simulink model "platoon1"  (R2023a)
settings: Solver=ode2  StartTime=0.0  StopTime=20  FixedStep=1/600  RelTol=1e-3  EnableMultiTasking=on
undefined symbols (not defined in the file or in its folder): HIL, qc_get_step_size
libraries: simulink x29, quarc_library x29, slpidlib x27, cstblocks x23, eeStairGenerator x1
(part 3 of 4)

== system platoon1/Controller8 ==
  PosPred : Inport
  PosEgo : Inport  Port=2
  d_ref : Inport  Port=3
  PosLead : Inport  Port=4
  i : Inport  Port=5
  Add : Sum  Inputs=+-
  Add1 : Sum  Inputs=-+
  Add2 : Sum
  Add3 : Sum  Inputs=+-
  Add4 : Sum  Inputs=-+
  Integrator : Integrator
  PID Controller : slpidlib/PID Controller  Controller=PID  Form=Parallel  TimeDomain=Continuous-time  UseExternalTs=off  SampleTime=-1  IntegratorMethod=Forward Euler  FilterMethod=Forward Euler  ControllerParametersSource=internal  P=0.33095280227445  I=0.0676054764431606  UseKiTs=off  D=0.347839718693587  N=40.6182647095365  UseFilter=on  TunerSelectOption=Transfer Function Based (PID Tuner App)  InitialConditionSource=internal  InitialConditionForIntegrator=0  InitialConditionForFilter=0  DifferentiatorICPrevScaledInput=0  ExternalReset=none  TrackingMode=off  Kt=1  LimitOutput=off  SatLimitsSource=internal  UpperSaturationLimit=inf  LowerSaturationLimit=-inf  LinearizeAsGain=on  AntiWindupMode=none  Kb=1  LimitIntegrator=off  UpperIntegratorSaturationLimit=inf  LowerIntegratorSaturationLimit=-inf  POutMin=[]  POutMax=[]  IOutMin=[]  IOutMax=[]  DOutMin=[]  DOutMax=[]  NOutMin=[]  NOutMax=[]  SumOutMin=[]  SumOutMax=[]  SaturationOutMin=[]  SaturationOutMax=[]  PParamMin=[]  PParamMax=[]  IParamMin=[]  IParamMax=[]  DParamMin=[]  DParamMax=[]  NParamMin=[]  NParamMax=[]  KbParamMin=[]  KbParamMax=[]  KtParamMin=[]  KtParamMax=[]  KbOutMin=[]  KbOutMax=[]  KtOutMin=[]  KtOutMax=[]  IntegratorOutMin=[]  IntegratorOutMax=[]  FilterOutMin=[]  FilterOutMax=[]  SumI1OutMin=[]  SumI1OutMax=[]  SumI2OutMin=[]  SumI2OutMax=[]  SumI3OutMin=[]  SumI3OutMax=[]  SumI4OutMin=[]  SumI4OutMax=[]  SumDOutMin=[]  SumDOutMax=[]  DifferentiatorOutMin=[]  DifferentiatorOutMax=[]  FilterDiffOutCoefMin=[]  FilterDiffOutCoefMax=[]  ReciprocalOutMin=[]  ReciprocalOutMax=[]  SumDenOutMin=[]  SumDenOutMax=[]  SumNumOutMin=[]  SumNumOutMax=[]  DivideOutMin=[]  DivideOutMax=[]  UdiffTsProdOutMin=[]  UdiffTsProdOutMax=[]  NTsProdOutMin=[]  NTsProdOutMax=[]  UintegralTsProdOutMin=[]  UintegralTsProdOutMax=[]  UngainTsProdOutMin=[]  UngainTsProdOutMax=[]  ClampingZeroOutDataTypeStr=Inherit: Inherit via back propagation  ClampingZeroOutMin=[]  ClampingZeroOutMax=[]  FilterDenConstantOutDataTypeStr=Inherit: Inherit via back propagation  FilterDenConstantOutMin=[]  FilterDenConstantOutMax=[]  PCopyOutDataTypeStr=Inherit: Inherit via back propagation  PCopyOutMin=[]  PCopyOutMax=[]  NCopyOutDataTypeStr=Inherit: Inherit via back propagation  NCopyOutMin=[]  NCopyOutMax=[]  IntegratorContinuousStateAttributes=''  IntegratorStateMustResolveToSignalObject=off  IntegratorRTWStateStorageClass=Auto  FilterContinuousStateAttributes=''  FilterStateMustResolveToSignalObject=off  FilterRTWStateStorageClass=Auto  ParallelPVariant=InternalParameters  IdealPVariant=Disabled  IVariant=InternalParameters  DVariant=InternalParameters  IntegratorVariant=Continuous  SatVariant=Disabled  AWVariant=Passthrough  PCopyVariant=Disabled  TRVariant=Disabled  FdbkBlocksVariant=Forward  IdealPFdbkVariant=Disabled  SatFdbkVariant=Disabled  DerivativeFilterVariant=ContFilter  NVariant=InternalParameters  NCopyVariant=Disabled  FilterICVariant=InternalICsFilter  IntegratorICVariant=InternalICs  ExternalResetVariant=Disabled  TRSumVariant=Passthrough  SumFdbkVariant=Disabled  SumVariant=Sum_PID  TsampFilterVariant=InternalTs  TsampNgainVariant=Passthrough  TsampIntegralVariant=Disabled_SignalSpec  ExternalSaturationOutDataTypeStr=Inherit: Same as second input
  PID Controller1 : slpidlib/PID Controller  Controller=PID  Form=Parallel  TimeDomain=Continuous-time  UseExternalTs=off  SampleTime=-1  IntegratorMethod=Forward Euler  FilterMethod=Forward Euler  ControllerParametersSource=internal  P=0.0689075408458366  I=0.00109879069900871  UseKiTs=off  D=0.960150912828831  N=312.36902011058  UseFilter=on  TunerSelectOption=Transfer Function Based (PID Tuner App)  InitialConditionSource=internal  InitialConditionForIntegrator=0  InitialConditionForFilter=0  DifferentiatorICPrevScaledInput=0  ExternalReset=none  TrackingMode=off  Kt=1  LimitOutput=off  SatLimitsSource=internal  UpperSaturationLimit=inf  LowerSaturationLimit=-inf  LinearizeAsGain=on  AntiWindupMode=none  Kb=1  LimitIntegrator=off  UpperIntegratorSaturationLimit=inf  LowerIntegratorSaturationLimit=-inf  POutMin=[]  POutMax=[]  IOutMin=[]  IOutMax=[]  DOutMin=[]  DOutMax=[]  NOutMin=[]  NOutMax=[]  SumOutMin=[]  SumOutMax=[]  SaturationOutMin=[]  SaturationOutMax=[]  PParamMin=[]  PParamMax=[]  IParamMin=[]  IParamMax=[]  DParamMin=[]  DParamMax=[]  NParamMin=[]  NParamMax=[]  KbParamMin=[]  KbParamMax=[]  KtParamMin=[]  KtParamMax=[]  KbOutMin=[]  KbOutMax=[]  KtOutMin=[]  KtOutMax=[]  IntegratorOutMin=[]  IntegratorOutMax=[]  FilterOutMin=[]  FilterOutMax=[]  SumI1OutMin=[]  SumI1OutMax=[]  SumI2OutMin=[]  SumI2OutMax=[]  SumI3OutMin=[]  SumI3OutMax=[]  SumI4OutMin=[]  SumI4OutMax=[]  SumDOutMin=[]  SumDOutMax=[]  DifferentiatorOutMin=[]  DifferentiatorOutMax=[]  FilterDiffOutCoefMin=[]  FilterDiffOutCoefMax=[]  ReciprocalOutMin=[]  ReciprocalOutMax=[]  SumDenOutMin=[]  SumDenOutMax=[]  SumNumOutMin=[]  SumNumOutMax=[]  DivideOutMin=[]  DivideOutMax=[]  UdiffTsProdOutMin=[]  UdiffTsProdOutMax=[]  NTsProdOutMin=[]  NTsProdOutMax=[]  UintegralTsProdOutMin=[]  UintegralTsProdOutMax=[]  UngainTsProdOutMin=[]  UngainTsProdOutMax=[]  ClampingZeroOutDataTypeStr=Inherit: Inherit via back propagation  ClampingZeroOutMin=[]  ClampingZeroOutMax=[]  FilterDenConstantOutDataTypeStr=Inherit: Inherit via back propagation  FilterDenConstantOutMin=[]  FilterDenConstantOutMax=[]  PCopyOutDataTypeStr=Inherit: Inherit via back propagation  PCopyOutMin=[]  PCopyOutMax=[]  NCopyOutDataTypeStr=Inherit: Inherit via back propagation  NCopyOutMin=[]  NCopyOutMax=[]  IntegratorContinuousStateAttributes=''  IntegratorStateMustResolveToSignalObject=off  IntegratorRTWStateStorageClass=Auto  FilterContinuousStateAttributes=''  FilterStateMustResolveToSignalObject=off  FilterRTWStateStorageClass=Auto  ParallelPVariant=InternalParameters  IdealPVariant=Disabled  IVariant=InternalParameters  DVariant=InternalParameters  IntegratorVariant=Continuous  SatVariant=Disabled  AWVariant=Passthrough  PCopyVariant=Disabled  TRVariant=Disabled  FdbkBlocksVariant=Forward  IdealPFdbkVariant=Disabled  SatFdbkVariant=Disabled  DerivativeFilterVariant=ContFilter  NVariant=InternalParameters  NCopyVariant=Disabled  FilterICVariant=InternalICsFilter  IntegratorICVariant=InternalICs  ExternalResetVariant=Disabled  TRSumVariant=Passthrough  SumFdbkVariant=Disabled  SumVariant=Sum_PID  TsampFilterVariant=InternalTs  TsampNgainVariant=Passthrough  TsampIntegralVariant=Disabled_SignalSpec  ExternalSaturationOutDataTypeStr=Inherit: Same as second input
  Product : Product
  Speed : Outport
  wires:
  PosPred/1 -> Add/1
  PosEgo/1 -> Add/2, Add3/2
  Add/1 -> Add1/2  "d_act"
  d_ref/1 -> Product/2, Add1/1
  Add1/1 -> PID Controller/1  "d_error_pred"
  Add2/1 -> Integrator/1
  PID Controller/1 -> Add2/2
  PosLead/1 -> Add3/1
  Add3/1 -> Add4/2  "d_act"
  Product/1 -> Add4/1
  i/1 -> Product/1
  Add4/1 -> PID Controller1/1  "d_error_lead"
  PID Controller1/1 -> Add2/1
  Integrator/1 -> Speed/1

== system platoon1/Controller9 ==
  PosPred : Inport
  PosEgo : Inport  Port=2
  d_ref : Inport  Port=3
  PosLead : Inport  Port=4
  i : Inport  Port=5
  Add : Sum  Inputs=+-
  Add1 : Sum  Inputs=-+
  Add2 : Sum
  Add3 : Sum  Inputs=+-
  Add4 : Sum  Inputs=-+
  Integrator : Integrator
  PID Controller : slpidlib/PID Controller  Controller=PID  Form=Parallel  TimeDomain=Continuous-time  UseExternalTs=off  SampleTime=-1  IntegratorMethod=Forward Euler  FilterMethod=Forward Euler  ControllerParametersSource=internal  P=0.33095280227445  I=0.0676054764431606  UseKiTs=off  D=0.347839718693587  N=40.6182647095365  UseFilter=on  TunerSelectOption=Transfer Function Based (PID Tuner App)  InitialConditionSource=internal  InitialConditionForIntegrator=0  InitialConditionForFilter=0  DifferentiatorICPrevScaledInput=0  ExternalReset=none  TrackingMode=off  Kt=1  LimitOutput=off  SatLimitsSource=internal  UpperSaturationLimit=inf  LowerSaturationLimit=-inf  LinearizeAsGain=on  AntiWindupMode=none  Kb=1  LimitIntegrator=off  UpperIntegratorSaturationLimit=inf  LowerIntegratorSaturationLimit=-inf  POutMin=[]  POutMax=[]  IOutMin=[]  IOutMax=[]  DOutMin=[]  DOutMax=[]  NOutMin=[]  NOutMax=[]  SumOutMin=[]  SumOutMax=[]  SaturationOutMin=[]  SaturationOutMax=[]  PParamMin=[]  PParamMax=[]  IParamMin=[]  IParamMax=[]  DParamMin=[]  DParamMax=[]  NParamMin=[]  NParamMax=[]  KbParamMin=[]  KbParamMax=[]  KtParamMin=[]  KtParamMax=[]  KbOutMin=[]  KbOutMax=[]  KtOutMin=[]  KtOutMax=[]  IntegratorOutMin=[]  IntegratorOutMax=[]  FilterOutMin=[]  FilterOutMax=[]  SumI1OutMin=[]  SumI1OutMax=[]  SumI2OutMin=[]  SumI2OutMax=[]  SumI3OutMin=[]  SumI3OutMax=[]  SumI4OutMin=[]  SumI4OutMax=[]  SumDOutMin=[]  SumDOutMax=[]  DifferentiatorOutMin=[]  DifferentiatorOutMax=[]  FilterDiffOutCoefMin=[]  FilterDiffOutCoefMax=[]  ReciprocalOutMin=[]  ReciprocalOutMax=[]  SumDenOutMin=[]  SumDenOutMax=[]  SumNumOutMin=[]  SumNumOutMax=[]  DivideOutMin=[]  DivideOutMax=[]  UdiffTsProdOutMin=[]  UdiffTsProdOutMax=[]  NTsProdOutMin=[]  NTsProdOutMax=[]  UintegralTsProdOutMin=[]  UintegralTsProdOutMax=[]  UngainTsProdOutMin=[]  UngainTsProdOutMax=[]  ClampingZeroOutDataTypeStr=Inherit: Inherit via back propagation  ClampingZeroOutMin=[]  ClampingZeroOutMax=[]  FilterDenConstantOutDataTypeStr=Inherit: Inherit via back propagation  FilterDenConstantOutMin=[]  FilterDenConstantOutMax=[]  PCopyOutDataTypeStr=Inherit: Inherit via back propagation  PCopyOutMin=[]  PCopyOutMax=[]  NCopyOutDataTypeStr=Inherit: Inherit via back propagation  NCopyOutMin=[]  NCopyOutMax=[]  IntegratorContinuousStateAttributes=''  IntegratorStateMustResolveToSignalObject=off  IntegratorRTWStateStorageClass=Auto  FilterContinuousStateAttributes=''  FilterStateMustResolveToSignalObject=off  FilterRTWStateStorageClass=Auto  ParallelPVariant=InternalParameters  IdealPVariant=Disabled  IVariant=InternalParameters  DVariant=InternalParameters  IntegratorVariant=Continuous  SatVariant=Disabled  AWVariant=Passthrough  PCopyVariant=Disabled  TRVariant=Disabled  FdbkBlocksVariant=Forward  IdealPFdbkVariant=Disabled  SatFdbkVariant=Disabled  DerivativeFilterVariant=ContFilter  NVariant=InternalParameters  NCopyVariant=Disabled  FilterICVariant=InternalICsFilter  IntegratorICVariant=InternalICs  ExternalResetVariant=Disabled  TRSumVariant=Passthrough  SumFdbkVariant=Disabled  SumVariant=Sum_PID  TsampFilterVariant=InternalTs  TsampNgainVariant=Passthrough  TsampIntegralVariant=Disabled_SignalSpec  ExternalSaturationOutDataTypeStr=Inherit: Same as second input
  PID Controller1 : slpidlib/PID Controller  Controller=PID  Form=Parallel  TimeDomain=Continuous-time  UseExternalTs=off  SampleTime=-1  IntegratorMethod=Forward Euler  FilterMethod=Forward Euler  ControllerParametersSource=internal  P=0.0689075408458366  I=0.00109879069900871  UseKiTs=off  D=0.960150912828831  N=312.36902011058  UseFilter=on  TunerSelectOption=Transfer Function Based (PID Tuner App)  InitialConditionSource=internal  InitialConditionForIntegrator=0  InitialConditionForFilter=0  DifferentiatorICPrevScaledInput=0  ExternalReset=none  TrackingMode=off  Kt=1  LimitOutput=off  SatLimitsSource=internal  UpperSaturationLimit=inf  LowerSaturationLimit=-inf  LinearizeAsGain=on  AntiWindupMode=none  Kb=1  LimitIntegrator=off  UpperIntegratorSaturationLimit=inf  LowerIntegratorSaturationLimit=-inf  POutMin=[]  POutMax=[]  IOutMin=[]  IOutMax=[]  DOutMin=[]  DOutMax=[]  NOutMin=[]  NOutMax=[]  SumOutMin=[]  SumOutMax=[]  SaturationOutMin=[]  SaturationOutMax=[]  PParamMin=[]  PParamMax=[]  IParamMin=[]  IParamMax=[]  DParamMin=[]  DParamMax=[]  NParamMin=[]  NParamMax=[]  KbParamMin=[]  KbParamMax=[]  KtParamMin=[]  KtParamMax=[]  KbOutMin=[]  KbOutMax=[]  KtOutMin=[]  KtOutMax=[]  IntegratorOutMin=[]  IntegratorOutMax=[]  FilterOutMin=[]  FilterOutMax=[]  SumI1OutMin=[]  SumI1OutMax=[]  SumI2OutMin=[]  SumI2OutMax=[]  SumI3OutMin=[]  SumI3OutMax=[]  SumI4OutMin=[]  SumI4OutMax=[]  SumDOutMin=[]  SumDOutMax=[]  DifferentiatorOutMin=[]  DifferentiatorOutMax=[]  FilterDiffOutCoefMin=[]  FilterDiffOutCoefMax=[]  ReciprocalOutMin=[]  ReciprocalOutMax=[]  SumDenOutMin=[]  SumDenOutMax=[]  SumNumOutMin=[]  SumNumOutMax=[]  DivideOutMin=[]  DivideOutMax=[]  UdiffTsProdOutMin=[]  UdiffTsProdOutMax=[]  NTsProdOutMin=[]  NTsProdOutMax=[]  UintegralTsProdOutMin=[]  UintegralTsProdOutMax=[]  UngainTsProdOutMin=[]  UngainTsProdOutMax=[]  ClampingZeroOutDataTypeStr=Inherit: Inherit via back propagation  ClampingZeroOutMin=[]  ClampingZeroOutMax=[]  FilterDenConstantOutDataTypeStr=Inherit: Inherit via back propagation  FilterDenConstantOutMin=[]  FilterDenConstantOutMax=[]  PCopyOutDataTypeStr=Inherit: Inherit via back propagation  PCopyOutMin=[]  PCopyOutMax=[]  NCopyOutDataTypeStr=Inherit: Inherit via back propagation  NCopyOutMin=[]  NCopyOutMax=[]  IntegratorContinuousStateAttributes=''  IntegratorStateMustResolveToSignalObject=off  IntegratorRTWStateStorageClass=Auto  FilterContinuousStateAttributes=''  FilterStateMustResolveToSignalObject=off  FilterRTWStateStorageClass=Auto  ParallelPVariant=InternalParameters  IdealPVariant=Disabled  IVariant=InternalParameters  DVariant=InternalParameters  IntegratorVariant=Continuous  SatVariant=Disabled  AWVariant=Passthrough  PCopyVariant=Disabled  TRVariant=Disabled  FdbkBlocksVariant=Forward  IdealPFdbkVariant=Disabled  SatFdbkVariant=Disabled  DerivativeFilterVariant=ContFilter  NVariant=InternalParameters  NCopyVariant=Disabled  FilterICVariant=InternalICsFilter  IntegratorICVariant=InternalICs  ExternalResetVariant=Disabled  TRSumVariant=Passthrough  SumFdbkVariant=Disabled  SumVariant=Sum_PID  TsampFilterVariant=InternalTs  TsampNgainVariant=Passthrough  TsampIntegralVariant=Disabled_SignalSpec  ExternalSaturationOutDataTypeStr=Inherit: Same as second input
  Product : Product
  Speed : Outport
  wires:
  PosPred/1 -> Add/1
  PosEgo/1 -> Add/2, Add3/2
  Add/1 -> Add1/2  "d_act"
  d_ref/1 -> Product/2, Add1/1
  Add1/1 -> PID Controller/1  "d_error_pred"
  Add2/1 -> Integrator/1
  PID Controller/1 -> Add2/2
  PosLead/1 -> Add3/1
  Add3/1 -> Add4/2  "d_act"
  Product/1 -> Add4/1
  i/1 -> Product/1
  Add4/1 -> PID Controller1/1  "d_error_lead"
  PID Controller1/1 -> Add2/1
  Integrator/1 -> Speed/1

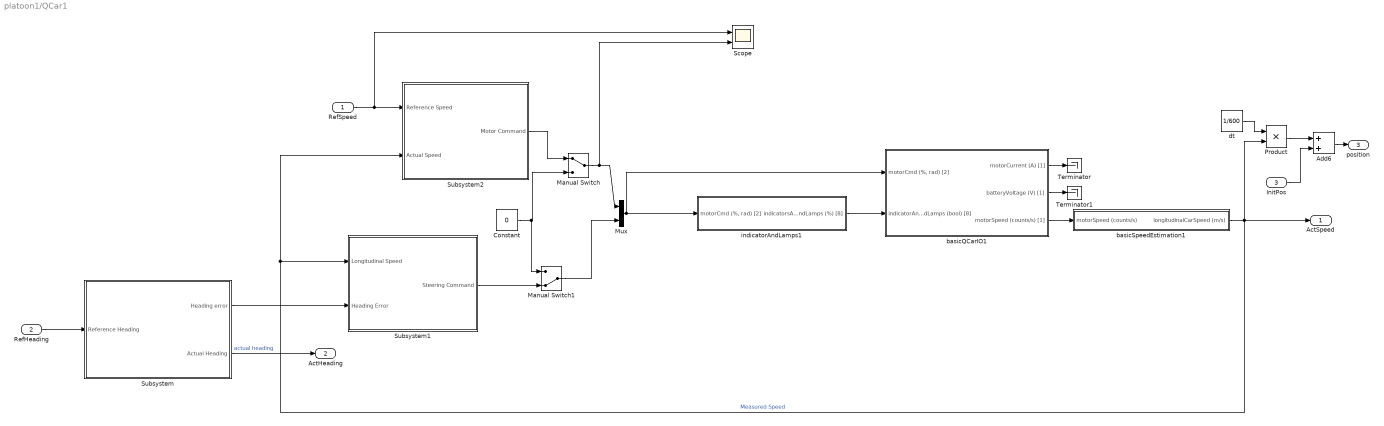
== system platoon1/QCar1 ==
  RefSpeed : Inport
  RefHeading : Inport  Port=2
  InitPos : Inport  Port=3
  Add6 : Sum
  Constant : Constant  Value=0
  Manual Switch : ManualSwitch
  Manual Switch1 : ManualSwitch  CurrentSetting=0
  Mux : Mux  Inputs=2
  Product : Product
  Scope : Scope  NumInputPorts=2
  Subsystem : Subsystem
  Subsystem1 : Subsystem
  Subsystem2 : Subsystem
  Terminator : Terminator
  Terminator1 : Terminator
  basicQCarIO1 : Subsystem
  basicSpeedEstimation1 : Subsystem
  dt : Constant  Value=1/600
  indicatorAndLamps1 : Subsystem
  ActSpeed : Outport
  ActHeading : Outport  Port=2
  position : Outport  Port=3
  wires:
  basicSpeedEstimation1/1(longitudinalCarSpeed (m/s)) -> Product/2, ActSpeed/1, Subsystem1/1(Longitudinal Speed), Subsystem2/2(Actual Speed)  "Measured Speed"
  Constant/1 -> Manual Switch/2, Manual Switch1/1
  Subsystem1/1(Steering Command) -> Manual Switch1/2
  Mux/1 -> basicQCarIO1/1("motorCmd (%, rad) [2]"), indicatorAndLamps1/1("motorCmd (%, rad) [2]")
  Subsystem2/1(Motor Command) -> Manual Switch/1
  RefSpeed/1 -> Scope/1, Subsystem2/1(Reference Speed)
  Manual Switch1/1 -> Mux/2
  Subsystem/2(Actual Heading) -> ActHeading/1  "actual heading"
  indicatorAndLamps1/1(indicatorsAndLamps (%) [8]) -> basicQCarIO1/2(indicatorAndLamps (bool) [8])
  RefHeading/1 -> Subsystem/1(Reference Heading)
  Manual Switch/1 -> Scope/2, Mux/1
  Subsystem/1(Heading error) -> Subsystem1/2(Heading Error)
  basicQCarIO1/3(motorSpeed (counts/s) [1]) -> basicSpeedEstimation1/1(motorSpeed (counts/s))
  basicQCarIO1/1(motorCurrent (A) [1]) -> Terminator/1
  basicQCarIO1/2(batteryVoltage (V) [1]) -> Terminator1/1
  InitPos/1 -> Add6/2
  Product/1 -> Add6/1
  Add6/1 -> position/1
  dt/1 -> Product/1

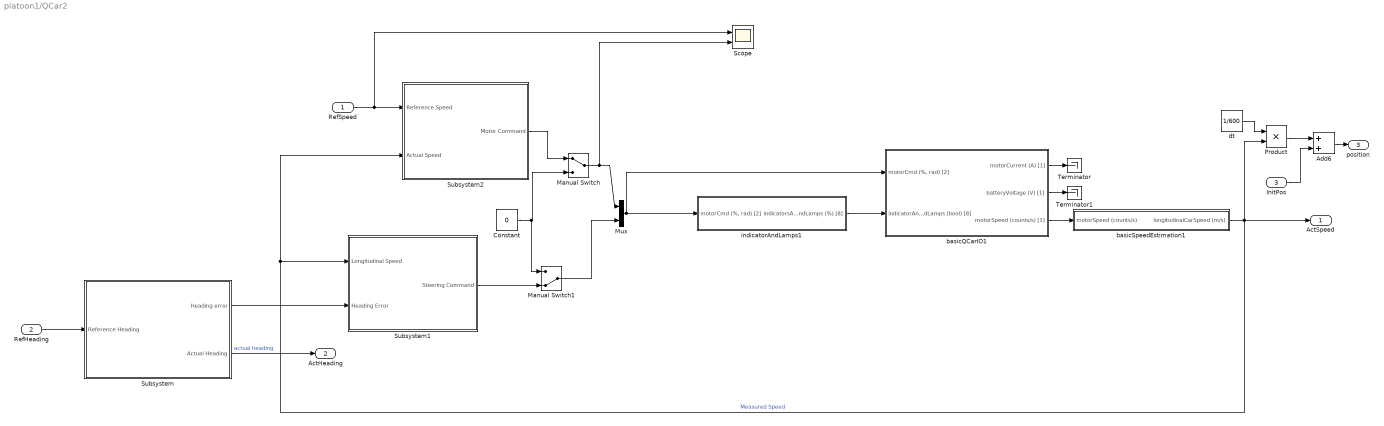
== system platoon1/QCar2 ==
  RefSpeed : Inport
  RefHeading : Inport  Port=2
  InitPos : Inport  Port=3
  Add6 : Sum
  Constant : Constant  Value=0
  Manual Switch : ManualSwitch
  Manual Switch1 : ManualSwitch  CurrentSetting=0
  Mux : Mux  Inputs=2
  Product : Product
  Scope : Scope  NumInputPorts=2
  Subsystem : Subsystem
  Subsystem1 : Subsystem
  Subsystem2 : Subsystem
  Terminator : Terminator
  Terminator1 : Terminator
  basicQCarIO1 : Subsystem
  basicSpeedEstimation1 : Subsystem
  dt : Constant  Value=1/600
  indicatorAndLamps1 : Subsystem
  ActSpeed : Outport
  ActHeading : Outport  Port=2
  position : Outport  Port=3
  wires:
  basicSpeedEstimation1/1(longitudinalCarSpeed (m/s)) -> Product/2, ActSpeed/1, Subsystem1/1(Longitudinal Speed), Subsystem2/2(Actual Speed)  "Measured Speed"
  Constant/1 -> Manual Switch/2, Manual Switch1/1
  Subsystem1/1(Steering Command) -> Manual Switch1/2
  Mux/1 -> basicQCarIO1/1("motorCmd (%, rad) [2]"), indicatorAndLamps1/1("motorCmd (%, rad) [2]")
  Subsystem2/1(Motor Command) -> Manual Switch/1
  RefSpeed/1 -> Scope/1, Subsystem2/1(Reference Speed)
  Manual Switch1/1 -> Mux/2
  Subsystem/2(Actual Heading) -> ActHeading/1  "actual heading"
  indicatorAndLamps1/1(indicatorsAndLamps (%) [8]) -> basicQCarIO1/2(indicatorAndLamps (bool) [8])
  RefHeading/1 -> Subsystem/1(Reference Heading)
  Manual Switch/1 -> Scope/2, Mux/1
  Subsystem/1(Heading error) -> Subsystem1/2(Heading Error)
  basicQCarIO1/3(motorSpeed (counts/s) [1]) -> basicSpeedEstimation1/1(motorSpeed (counts/s))
  basicQCarIO1/1(motorCurrent (A) [1]) -> Terminator/1
  basicQCarIO1/2(batteryVoltage (V) [1]) -> Terminator1/1
  InitPos/1 -> Add6/2
  Product/1 -> Add6/1
  Add6/1 -> position/1
  dt/1 -> Product/1

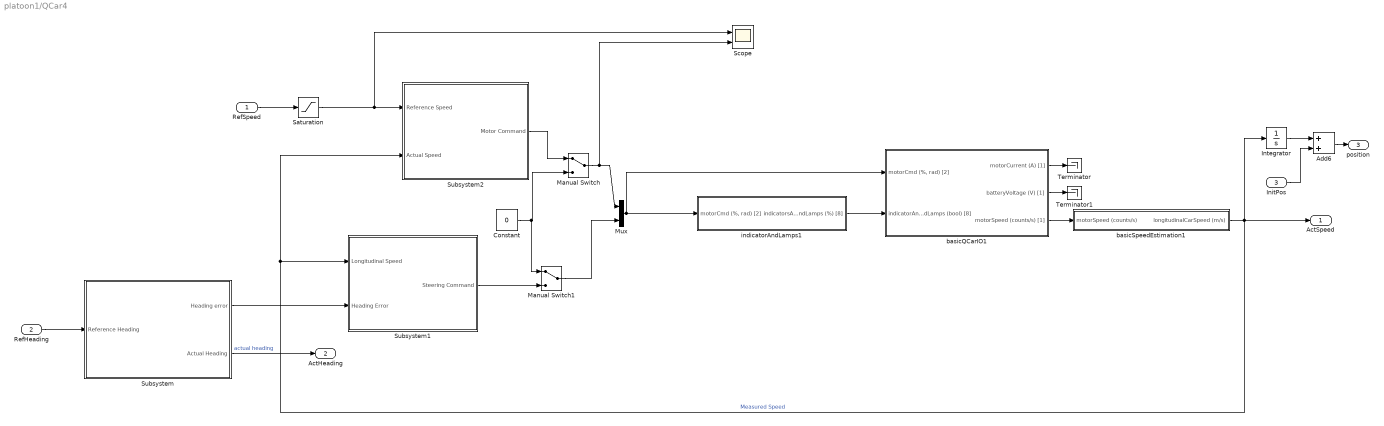
== system platoon1/QCar4 ==
  RefSpeed : Inport
  RefHeading : Inport  Port=2
  InitPos : Inport  Port=3
  Add6 : Sum
  Constant : Constant  Value=0
  Integrator : Integrator
  Manual Switch : ManualSwitch
  Manual Switch1 : ManualSwitch
  Mux : Mux  Inputs=2
  Saturation : Saturate  UpperLimit=0.6  LowerLimit=-0.6
  Scope : Scope  NumInputPorts=2
  Subsystem : Subsystem
  Subsystem1 : Subsystem
  Subsystem2 : Subsystem
  Terminator : Terminator
  Terminator1 : Terminator
  basicQCarIO1 : Subsystem
  basicSpeedEstimation1 : Subsystem
  indicatorAndLamps1 : Subsystem
  ActSpeed : Outport
  ActHeading : Outport  Port=2
  position : Outport  Port=3
  wires:
  basicSpeedEstimation1/1(longitudinalCarSpeed (m/s)) -> Integrator/1, ActSpeed/1, Subsystem1/1(Longitudinal Speed), Subsystem2/2(Actual Speed)  "Measured Speed"
  Constant/1 -> Manual Switch/2, Manual Switch1/1
  Subsystem1/1(Steering Command) -> Manual Switch1/2
  Mux/1 -> basicQCarIO1/1("motorCmd (%, rad) [2]"), indicatorAndLamps1/1("motorCmd (%, rad) [2]")
  Subsystem2/1(Motor Command) -> Manual Switch/1
  RefSpeed/1 -> Saturation/1
  Manual Switch1/1 -> Mux/2
  Subsystem/2(Actual Heading) -> ActHeading/1  "actual heading"
  indicatorAndLamps1/1(indicatorsAndLamps (%) [8]) -> basicQCarIO1/2(indicatorAndLamps (bool) [8])
  RefHeading/1 -> Subsystem/1(Reference Heading)
  Manual Switch/1 -> Scope/2, Mux/1
  Subsystem/1(Heading error) -> Subsystem1/2(Heading Error)
  basicQCarIO1/3(motorSpeed (counts/s) [1]) -> basicSpeedEstimation1/1(motorSpeed (counts/s))
  basicQCarIO1/1(motorCurrent (A) [1]) -> Terminator/1
  basicQCarIO1/2(batteryVoltage (V) [1]) -> Terminator1/1
  InitPos/1 -> Add6/2
  Integrator/1 -> Add6/1
  Add6/1 -> position/1
  Saturation/1 -> Scope/1, Subsystem2/1(Reference Speed)

== system platoon1/Virtual Car (TF) ==
  RefSpeed : Inport
  InitPos : Inport  Port=2
  Add6 : Sum
  Integrator : Integrator
  TF model : cstblocks/LTI System  sys=G4  IC=[]
  position : Outport
  speed : Outport  Port=2
  wires:
  Integrator/1 -> Add6/1
  RefSpeed/1 -> TF model/1
  InitPos/1 -> Add6/2
  TF model/1 -> Integrator/1, speed/1  "vel0"
  Add6/1 -> position/1

== system platoon1/Virtual Car (TF)1 ==
  RefSpeed : Inport
  InitPos : Inport  Port=2
  Add6 : Sum
  Integrator : Integrator
  TF model : cstblocks/LTI System  sys=G  IC=[]
  position : Outport
  speed : Outport  Port=2
  wires:
  Integrator/1 -> Add6/1
  RefSpeed/1 -> TF model/1
  InitPos/1 -> Add6/2
  TF model/1 -> Integrator/1, speed/1  "vel0"
  Add6/1 -> position/1

== system platoon1/Virtual Car (TF)10 ==
  RefSpeed : Inport
  InitPos : Inport  Port=2
  Add6 : Sum
  Integrator : Integrator
  TF model : cstblocks/LTI System  sys=G4  IC=[]
  position : Outport
  speed : Outport  Port=2
  wires:
  Integrator/1 -> Add6/1
  RefSpeed/1 -> TF model/1
  InitPos/1 -> Add6/2
  TF model/1 -> Integrator/1, speed/1  "vel0"
  Add6/1 -> position/1

== system platoon1/Virtual Car (TF)11 ==
  RefSpeed : Inport
  InitPos : Inport  Port=2
  Add6 : Sum
  Integrator : Integrator
  TF model : cstblocks/LTI System  sys=G4  IC=[]
  position : Outport
  speed : Outport  Port=2
  wires:
  Integrator/1 -> Add6/1
  RefSpeed/1 -> TF model/1
  InitPos/1 -> Add6/2
  TF model/1 -> Integrator/1, speed/1  "vel0"
  Add6/1 -> position/1

== system platoon1/Virtual Car (TF)12 ==
  RefSpeed : Inport
  InitPos : Inport  Port=2
  Add6 : Sum
  Integrator : Integrator
  TF model : cstblocks/LTI System  sys=G4  IC=[]
  position : Outport
  speed : Outport  Port=2
  wires:
  Integrator/1 -> Add6/1
  RefSpeed/1 -> TF model/1
  InitPos/1 -> Add6/2
  TF model/1 -> Integrator/1, speed/1  "vel0"
  Add6/1 -> position/1

== system platoon1/Virtual Car (TF)13 ==
  RefSpeed : Inport
  InitPos : Inport  Port=2
  Add6 : Sum
  Integrator : Integrator
  TF model : cstblocks/LTI System  sys=G4  IC=[]
  position : Outport
  speed : Outport  Port=2
  wires:
  Integrator/1 -> Add6/1
  RefSpeed/1 -> TF model/1
  InitPos/1 -> Add6/2
  TF model/1 -> Integrator/1, speed/1  "vel0"
  Add6/1 -> position/1

== system platoon1/Virtual Car (TF)14 ==
  RefSpeed : Inport
  InitPos : Inport  Port=2
  Add6 : Sum
  Integrator : Integrator
  TF model : cstblocks/LTI System  sys=G4  IC=[]
  position : Outport
  speed : Outport  Port=2
  wires:
  Integrator/1 -> Add6/1
  RefSpeed/1 -> TF model/1
  InitPos/1 -> Add6/2
  TF model/1 -> Integrator/1, speed/1  "vel0"
  Add6/1 -> position/1

== system platoon1/Virtual Car (TF)15 ==
  RefSpeed : Inport
  InitPos : Inport  Port=2
  Add6 : Sum
  Integrator : Integrator
  TF model : cstblocks/LTI System  sys=G4  IC=[]
  position : Outport
  speed : Outport  Port=2
  wires:
  Integrator/1 -> Add6/1
  RefSpeed/1 -> TF model/1
  InitPos/1 -> Add6/2
  TF model/1 -> Integrator/1, speed/1  "vel0"
  Add6/1 -> position/1

== system platoon1/Virtual Car (TF)16 ==
  RefSpeed : Inport
  InitPos : Inport  Port=2
  Add6 : Sum
  Integrator : Integrator
  TF model : cstblocks/LTI System  sys=G  IC=[]
  position : Outport
  speed : Outport  Port=2
  wires:
  Integrator/1 -> Add6/1
  RefSpeed/1 -> TF model/1
  InitPos/1 -> Add6/2
  TF model/1 -> Integrator/1, speed/1  "vel0"
  Add6/1 -> position/1

== system platoon1/Virtual Car (TF)17 ==
  RefSpeed : Inport
  InitPos : Inport  Port=2
  Add6 : Sum
  Integrator : Integrator
  TF model : cstblocks/LTI System  sys=G  IC=[]
  position : Outport
  speed : Outport  Port=2
  wires:
  Integrator/1 -> Add6/1
  TF model/1 -> Integrator/1, speed/1  "vel0"
  RefSpeed/1 -> TF model/1
  Add6/1 -> position/1
  InitPos/1 -> Add6/2

== system platoon1/Virtual Car (TF)18 ==
  RefSpeed : Inport
  InitPos : Inport  Port=2
  Add6 : Sum
  Integrator : Integrator
  TF model : cstblocks/LTI System  sys=G  IC=[]
  position : Outport
  speed : Outport  Port=2
  wires:
  Integrator/1 -> Add6/1
  TF model/1 -> Integrator/1, speed/1  "vel0"
  RefSpeed/1 -> TF model/1
  Add6/1 -> position/1
  InitPos/1 -> Add6/2

== system platoon1/Virtual Car (TF)19 ==
  RefSpeed : Inport
  InitPos : Inport  Port=2
  Add6 : Sum
  Integrator : Integrator
  TF model : cstblocks/LTI System  sys=G4  IC=[]
  position : Outport
  speed : Outport  Port=2
  wires:
  Integrator/1 -> Add6/1
  TF model/1 -> Integrator/1, speed/1  "vel0"
  RefSpeed/1 -> TF model/1
  Add6/1 -> position/1
  InitPos/1 -> Add6/2

== system platoon1/Virtual Car (TF)2 ==
  RefSpeed : Inport
  InitPos : Inport  Port=2
  Add6 : Sum
  Integrator : Integrator
  TF model : cstblocks/LTI System  sys=G  IC=[]
  position : Outport
  speed : Outport  Port=2
  wires:
  Integrator/1 -> Add6/1
  RefSpeed/1 -> TF model/1
  InitPos/1 -> Add6/2
  TF model/1 -> Integrator/1, speed/1  "vel0"
  Add6/1 -> position/1

== system platoon1/Virtual Car (TF)20 ==
  RefSpeed : Inport
  InitPos : Inport  Port=2
  Add6 : Sum
  Integrator : Integrator
  TF model : cstblocks/LTI System  sys=G4  IC=[]
  position : Outport
  speed : Outport  Port=2
  wires:
  Integrator/1 -> Add6/1
  TF model/1 -> Integrator/1, speed/1  "vel0"
  RefSpeed/1 -> TF model/1
  Add6/1 -> position/1
  InitPos/1 -> Add6/2

== system platoon1/Virtual Car (TF)21 ==
  RefSpeed : Inport
  InitPos : Inport  Port=2
  Add6 : Sum
  Integrator : Integrator
  TF model : cstblocks/LTI System  sys=G  IC=[]
  position : Outport
  speed : Outport  Port=2
  wires:
  Integrator/1 -> Add6/1
  TF model/1 -> Integrator/1, speed/1  "vel0"
  RefSpeed/1 -> TF model/1
  Add6/1 -> position/1
  InitPos/1 -> Add6/2

== system platoon1/Virtual Car (TF)22 ==
  RefSpeed : Inport
  InitPos : Inport  Port=2
  Add6 : Sum
  Integrator : Integrator
  TF model : cstblocks/LTI System  sys=G4  IC=[]
  position : Outport
  speed : Outport  Port=2
  wires:
  Integrator/1 -> Add6/1
  RefSpeed/1 -> TF model/1
  InitPos/1 -> Add6/2
  TF model/1 -> Integrator/1, speed/1  "vel0"
  Add6/1 -> position/1

== system platoon1/Virtual Car (TF)3 ==
  RefSpeed : Inport
  InitPos : Inport  Port=2
  Add6 : Sum
  Integrator : Integrator
  TF model : cstblocks/LTI System  sys=G  IC=[]
  position : Outport
  speed : Outport  Port=2
  wires:
  Integrator/1 -> Add6/1
  TF model/1 -> Integrator/1, speed/1  "vel0"
  RefSpeed/1 -> TF model/1
  Add6/1 -> position/1
  InitPos/1 -> Add6/2

== system platoon1/Virtual Car (TF)4 ==
  RefSpeed : Inport
  InitPos : Inport  Port=2
  Add6 : Sum
  Integrator : Integrator
  TF model : cstblocks/LTI System  sys=G  IC=[]
  position : Outport
  speed : Outport  Port=2
  wires:
  Integrator/1 -> Add6/1
  TF model/1 -> Integrator/1, speed/1  "vel0"
  RefSpeed/1 -> TF model/1
  Add6/1 -> position/1
  InitPos/1 -> Add6/2

== system platoon1/Virtual Car (TF)5 ==
  RefSpeed : Inport
  InitPos : Inport  Port=2
  Add6 : Sum
  Integrator : Integrator
  TF model : cstblocks/LTI System  sys=G  IC=[]
  position : Outport
  speed : Outport  Port=2
  wires:
  Integrator/1 -> Add6/1
  TF model/1 -> Integrator/1, speed/1  "vel0"
  RefSpeed/1 -> TF model/1
  Add6/1 -> position/1
  InitPos/1 -> Add6/2

== system platoon1/Virtual Car (TF)6 ==
  RefSpeed : Inport
  InitPos : Inport  Port=2
  Add6 : Sum
  Integrator : Integrator
  TF model : cstblocks/LTI System  sys=G  IC=[]
  position : Outport
  speed : Outport  Port=2
  wires:
  Integrator/1 -> Add6/1
  TF model/1 -> Integrator/1, speed/1  "vel0"
  RefSpeed/1 -> TF model/1
  Add6/1 -> position/1
  InitPos/1 -> Add6/2

== system platoon1/Virtual Car (TF)7 ==
  RefSpeed : Inport
  InitPos : Inport  Port=2
  Add6 : Sum
  Integrator : Integrator
  TF model : cstblocks/LTI System  sys=G  IC=[]
  position : Outport
  speed : Outport  Port=2
  wires:
  Integrator/1 -> Add6/1
  TF model/1 -> Integrator/1, speed/1  "vel0"
  RefSpeed/1 -> TF model/1
  Add6/1 -> position/1
  InitPos/1 -> Add6/2

== system platoon1/Virtual Car (TF)8 ==
  RefSpeed : Inport
  InitPos : Inport  Port=2
  Add6 : Sum
  Integrator : Integrator
  TF model : cstblocks/LTI System  sys=G  IC=[]
  position : Outport
  speed : Outport  Port=2
  wires:
  Integrator/1 -> Add6/1
  RefSpeed/1 -> TF model/1
  InitPos/1 -> Add6/2
  TF model/1 -> Integrator/1, speed/1  "vel0"
  Add6/1 -> position/1

== system platoon1/Virtual Car (TF)9 ==
  RefSpeed : Inport
  InitPos : Inport  Port=2
  Add6 : Sum
  Integrator : Integrator
  TF model : cstblocks/LTI System  sys=G4  IC=[]
  position : Outport
  speed : Outport  Port=2
  wires:
  Integrator/1 -> Add6/1
  RefSpeed/1 -> TF model/1
  InitPos/1 -> Add6/2
  TF model/1 -> Integrator/1, speed/1  "vel0"
  Add6/1 -> position/1

== system platoon1/QCar1/Subsystem ==
  note: Adjust your filter to find a compromise
      | between noise filtering and bandwidth
  note: This will auto-calibrate the drift compensation
      | on each run. Ignore the warm up samples
      | then calculate the offset for the next set of samples.
      | If the offset value is consistent in your operating
      | environment, this can be replaced with the measured
      | constant.
  note: Select the Yaw axis
  note: Integrate the angular velocity to
      | get your heading.
  note: Examing the board-specific options
      | in the HIL Initialize (found in the Basic
      | QCar IO block) for additional filter
      | and bandwidth options.
  Reference Heading : Inport
  Ignore initial samples for sensor warmup : Constant  Value=1000
  Integrator : Integrator  ExternalReset=rising
  MATLAB Function : MATLAB Function  TreatAsAtomicUnit=on
  Number of samples for drift compensation : Constant  Value=1000
  Selector : Selector  InputPortWidth=3  IndexOptions=Index vector (dialog)  Indices=[3]  OutputSizes=1
  Sum1 : Sum  Inputs=|+-
  Sum2 : Sum  Inputs=+-|
  Transfer Fcn : TransferFcn  Numerator=[10]  Denominator=[1 10]
  readIMU Module : Subsystem
  Heading error : Outport
  Actual Heading : Outport  Port=2
  wires:
  readIMU Module/1(gyroscope (rad/s) [3]) -> Selector/1
  Number of samples for drift compensation/1 -> MATLAB Function/2(samples)
  Integrator/1 -> Actual Heading/1, Sum2/2
  Transfer Fcn/1 -> Sum1/1, MATLAB Function/1(u)
  Selector/1 -> Transfer Fcn/1
  Ignore initial samples for sensor warmup/1 -> MATLAB Function/3(startup_samples)
  Sum1/1 -> Integrator/1
  MATLAB Function/2(ready) -> Integrator/2
  Sum2/1 -> Heading error/1
  MATLAB Function/1(offset) -> Sum1/2
  Reference Heading/1 -> Sum2/1

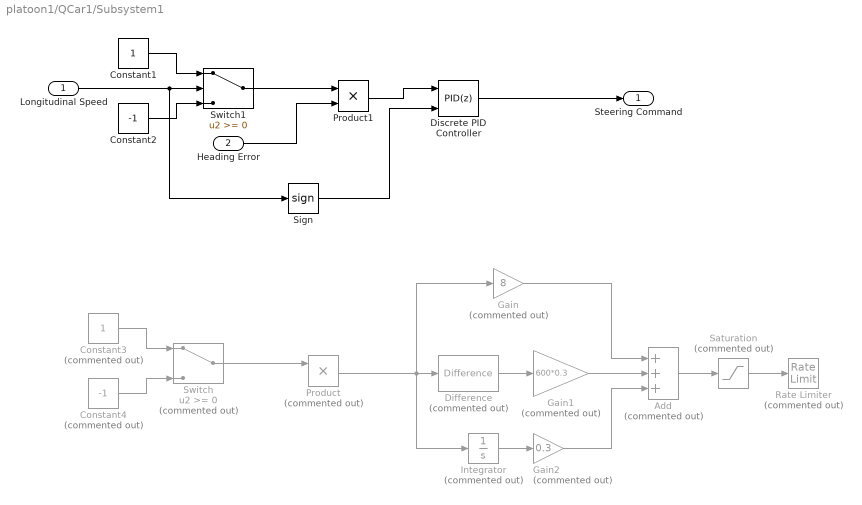
== system platoon1/QCar1/Subsystem1 ==
  Longitudinal Speed : Inport
  Heading Error : Inport  Port=2
  Add : Sum  Commented=on  Inputs=+++
  Constant1 : Constant
  Constant2 : Constant  Value=-1
  Constant3 : Constant  Commented=on
  Constant4 : Constant  Commented=on  Value=-1
  Difference : simulink/Discrete/Difference  Commented=on  ICPrevInput=0.0  OutMin=[]  OutMax=[]  OutDataType=fixdt(1, 16)  OutScaling=2^-10  DoSatur=off
  Discrete PID Controller : slpidlib/PID Controller  Controller=PID  Form=Parallel  TimeDomain=Discrete-time  UseExternalTs=off  SampleTime=-1  IntegratorMethod=Forward Euler  FilterMethod=Forward Euler  ControllerParametersSource=internal  P=1  I=1  UseKiTs=off  D=0.1  N=100  UseFilter=on  TunerSelectOption=Transfer Function Based (PID Tuner App)  InitialConditionSource=internal  InitialConditionForIntegrator=0  InitialConditionForFilter=0  DifferentiatorICPrevScaledInput=0  ExternalReset=either  TrackingMode=off  Kt=1  LimitOutput=on  SatLimitsSource=internal  UpperSaturationLimit=0.5  LowerSaturationLimit=-0.5  LinearizeAsGain=on  AntiWindupMode=clamping  Kb=1  LimitIntegrator=off  UpperIntegratorSaturationLimit=inf  LowerIntegratorSaturationLimit=-inf  POutMin=[]  POutMax=[]  IOutMin=[]  IOutMax=[]  DOutMin=[]  DOutMax=[]  NOutMin=[]  NOutMax=[]  SumOutMin=[]  SumOutMax=[]  SaturationOutMin=[]  SaturationOutMax=[]  PParamMin=[]  PParamMax=[]  IParamMin=[]  IParamMax=[]  DParamMin=[]  DParamMax=[]  NParamMin=[]  NParamMax=[]  KbParamMin=[]  KbParamMax=[]  KtParamMin=[]  KtParamMax=[]  KbOutMin=[]  KbOutMax=[]  KtOutMin=[]  KtOutMax=[]  IntegratorOutMin=[]  IntegratorOutMax=[]  FilterOutMin=[]  FilterOutMax=[]  SumI1OutMin=[]  SumI1OutMax=[]  SumI2OutMin=[]  SumI2OutMax=[]  SumI3OutMin=[]  SumI3OutMax=[]  SumI4OutMin=[]  SumI4OutMax=[]  SumDOutMin=[]  SumDOutMax=[]  DifferentiatorOutMin=[]  DifferentiatorOutMax=[]  FilterDiffOutCoefMin=[]  FilterDiffOutCoefMax=[]  ReciprocalOutMin=[]  ReciprocalOutMax=[]  SumDenOutMin=[]  SumDenOutMax=[]  SumNumOutMin=[]  SumNumOutMax=[]  DivideOutMin=[]  DivideOutMax=[]  UdiffTsProdOutMin=[]  UdiffTsProdOutMax=[]  NTsProdOutMin=[]  NTsProdOutMax=[]  UintegralTsProdOutMin=[]  UintegralTsProdOutMax=[]  UngainTsProdOutMin=[]  UngainTsProdOutMax=[]  ClampingZeroOutDataTypeStr=Inherit: Inherit via back propagation  ClampingZeroOutMin=[]  ClampingZeroOutMax=[]  FilterDenConstantOutDataTypeStr=Inherit: Inherit via back propagation  FilterDenConstantOutMin=[]  FilterDenConstantOutMax=[]  PCopyOutDataTypeStr=Inherit: Inherit via back propagation  PCopyOutMin=[]  PCopyOutMax=[]  NCopyOutDataTypeStr=Inherit: Inherit via back propagation  NCopyOutMin=[]  NCopyOutMax=[]  IntegratorContinuousStateAttributes=''  IntegratorStateMustResolveToSignalObject=off  IntegratorRTWStateStorageClass=Auto  FilterContinuousStateAttributes=''  FilterStateMustResolveToSignalObject=off  FilterRTWStateStorageClass=Auto  ParallelPVariant=InternalParameters  IdealPVariant=Disabled  IVariant=InternalParameters  DVariant=InternalParameters  IntegratorVariant=Discrete  SatVariant=Enabled  AWVariant=DiscClampingParallel  PCopyVariant=Disabled  TRVariant=Disabled  FdbkBlocksVariant=Forward  IdealPFdbkVariant=Disabled  SatFdbkVariant=Disabled  DerivativeFilterVariant=ForwardEulerFilter  NVariant=InternalParameters  NCopyVariant=Disabled  FilterICVariant=InternalICsFilter  IntegratorICVariant=InternalICs  ExternalResetVariant=ExternalReset  TRSumVariant=Passthrough  SumFdbkVariant=Disabled  SumVariant=Sum_PID  TsampFilterVariant=InternalTs  TsampNgainVariant=Passthrough  TsampIntegralVariant=Disabled_SignalSpec  ExternalSaturationOutDataTypeStr=Inherit: Same as second input
  Gain : Gain  Commented=on  Gain=8
  Gain1 : Gain  Commented=on  Gain=600*0.3
  Gain2 : Gain  Commented=on  Gain=0.3
  Integrator : Integrator  Commented=on  LimitOutput=on  UpperSaturationLimit=0.4  LowerSaturationLimit=-0.4
  Product : Product  Commented=on
  Product1 : Product
  Rate Limiter : RateLimiter  Commented=on  RisingSlewLimit=0.3  FallingSlewLimit=-0.3  SampleTimeMode=inherited
  Saturation : Saturate  Commented=on
  Sign : Signum
  Switch : Switch  Commented=on  SaturateOnIntegerOverflow=off  InputSameDT=off
  Switch1 : Switch  SaturateOnIntegerOverflow=off  InputSameDT=off
  Steering Command : Outport
  wires:
  Constant3/1 -> Switch/1
  Switch/1 -> Product/1
  Product/1 -> Integrator/1, Difference/1, Gain/1
  Constant4/1 -> Switch/3
  Difference/1 -> Gain1/1
  Gain1/1 -> Add/2
  Add/1 -> Saturation/1
  Gain/1 -> Add/1
  Integrator/1 -> Gain2/1
  Gain2/1 -> Add/3
  Saturation/1 -> Rate Limiter/1
  Constant2/1 -> Switch1/3
  Constant1/1 -> Switch1/1
  Switch1/1 -> Product1/1
  Heading Error/1 -> Product1/2
  Longitudinal Speed/1 -> Sign/1, Switch1/2
  Product1/1 -> Discrete PID Controller/1
  Discrete PID Controller/1 -> Steering Command/1
  Sign/1 -> Discrete PID Controller/2

== system platoon1/QCar1/Subsystem2 ==
  note: Feedback
  note: Feedforward
  Reference Speed : Inport
  Actual Speed : Inport  Port=2
  Add : Sum
  Add1 : Sum
  Compare To Zero : simulink/Logic and Bit Operations/Compare To Zero  relop===  OutDataTypeStr=boolean
  Integrator1 : Integrator  ExternalReset=either  LimitOutput=on  UpperSaturationLimit=0.4  LowerSaturationLimit=-0.4
  Kff (% / m/s) : Gain  Gain=0.1
  "Ki (% / m) " : Gain
  Kp (% / m/s) : Gain  Gain=0.3
  Saturation : Saturate  UpperLimit=1  LowerLimit=-1
  Sum : Sum  Inputs=|+-
  command saturation : Saturate  UpperLimit=5  LowerLimit=-5
  Motor Command : Outport
  wires:
  Compare To Zero/1 -> Integrator1/2
  Kp (% / m/s)/1 -> Add/1
  "Ki (% / m) "/1 -> Integrator1/1
  command saturation/1 -> Kff (% / m/s)/1, Compare To Zero/1, Sum/1  "desired"
  Kff (% / m/s)/1 -> Add1/1
  Integrator1/1 -> Add/2
  Sum/1 -> "Ki (% / m) "/1, Kp (% / m/s)/1
  Reference Speed/1 -> command saturation/1
  Add/1 -> Add1/2
  Add1/1 -> Saturation/1
  Actual Speed/1 -> Sum/2
  Saturation/1 -> Motor Command/1

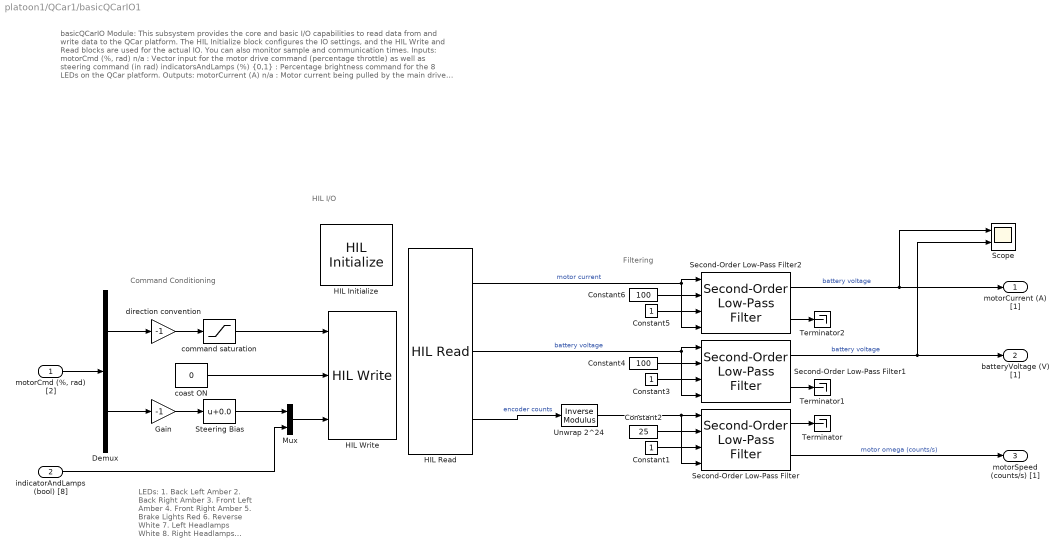
== system platoon1/QCar1/basicQCarIO1 ==
  note: Filtering
  note: basicQCarIO Module:
      |
      | This subsystem provides the core and basic I/O capabilities to read data from and write data to the QCar platform. The HIL Initialize block configures the IO settings, and the HIL Write and Read blocks are used for the actual IO. You can also monitor sample and communication times.
      |
      | Inputs:
      | motorCmd (%, rad) n/a : Vector input for the motor drive command (percentage throttle) as well as steering command (in rad)
      | indicatorsAndLamps (%) {0,1} : Percentage brightness command for the 8 LEDs on the QCar platform.
      |
      | Outputs:
      | motorCurrent (A) n/a : Motor current being pulled by the main drive motor
      | batteryVoltage (V) {0, 12.6} : Current battery voltage reading
      | motorSpeed (counts/s) n/a : Drive motor speed measured using an encoder (do not confuse with wheel speed as this measurement is at the drive shaft)
  note: Command Conditioning
  note: HIL I/O
  note: LEDs:
      | 1. Back Left Amber
      | 2. Back Right Amber
      | 3. Front Left Amber
      | 4. Front Right Amber
      | 5. Brake Lights Red
      | 6. Reverse White
      | 7. Left Headlamps White
      | 8. Right Headlamps White
  "motorCmd (%, rad) [2]" : Inport
  indicatorAndLamps (bool) [8] : Inport  Port=2
  Constant1 : Constant
  Constant2 : Constant  Value=25
  Constant3 : Constant
  Constant4 : Constant  Value=100
  Constant5 : Constant
  Constant6 : Constant  Value=100
  Demux : Demux  Outputs=2
  Gain : Gain  Gain=-1
  HIL Initialize : quarc_library/Data Acquisition/Generic/Configuration/HIL Initialize  object_name=HIL-2  board_type=qcar  board_number=0  board_options=gyro_fs=250;gyro_rate=64;accel_fs=2;accel_rate=62.5;mag_rate=20;mag_xy=47;mag_z=83;enc1_dir=0;enc2_dir=0;enc3_dir=0;enc4_dir=0;pwm1_dshot=0;pwm2_dshot=0;pwm3_dshot=0;pwm4_dshot=0;pwm5_dshot=0;pwm6_dshot=0;pwm7_dshot=0;steer_bias=0.05;motor_limit=0.3;  exclusive=off  active=on  hardware_clocks=[]  clock_modes=[]  initial_clock_frequencies=[]  set_clock_params_at_start=off  set_clock_params_at_switch_in=off  set_clock_frequencies_at_start=off  set_clock_frequencies_at_switch_in=off  analog_input_channels=[0:6]  analog_input_configurations=[]  analog_input_maximums=[3.3]  analog_input_minimums=[0]  set_analog_input_params_at_start=off  set_analog_input_params_at_switch_in=off  analog_output_channels=[]  analog_output_maximums=[]  analog_output_minimums=[]  initial_analog_outputs=[]  final_analog_outputs=[]  watchdog_analog_outputs=[]  set_analog_output_params_at_start=off  set_analog_output_params_at_switch_in=off  set_analog_outputs_at_start=off  set_analog_outputs_at_switch_in=off  set_analog_outputs_at_terminate=off  set_analog_outputs_at_switch_out=off  set_analog_outputs_on_watchdog=off  digital_input_channels=[24:43]  digital_output_channels=[40]  digital_output_configuration=[]  initial_digital_outputs=[0]  final_digital_outputs=[1]  watchdog_digital_outputs=[]  set_digital_output_params_at_start=off  set_digital_output_params_at_switch_in=off  set_digital_outputs_at_start=on  set_digital_outputs_at_switch_in=off  set_digital_outputs_at_terminate=on  set_digital_outputs_at_switch_out=off  set_digital_outputs_on_watchdog=off  encoder_channels=[0:4]  quadrature=[4 4]  encoder_filter_frequency=100e6/1  initial_encoder_counts=[0]  set_encoder_params_at_start=on  set_encoder_params_at_switch_in=off  set_encoder_counts_at_start=on  set_encoder_counts_at_switch_in=off  pwm_channels=[0:7]  pwm_modes=[0 0]  pwm_frequency=150e6/4096  pwm_configuration=[0]  pwm_alignment=[0]  pwm_polarity=[1]  pwm_leading_deadband=[]  pwm_trailing_deadband=[]  initial_pwm_outputs=[0]  final_pwm_outputs=[0]  watchdog_pwm_outputs=[0]  set_pwm_params_at_start=on  set_pwm_params_at_switch_in=off  set_pwm_outputs_at_start=on  set_pwm_outputs_at_switch_in=off  set_pwm_outputs_at_terminate=on  set_pwm_outputs_at_switch_out=off  set_pwm_outputs_on_watchdog=off  other_output_channels=[1000, 11000:11011]  initial_other_outputs=[0]  final_other_outputs=[0]  watchdog_other_outputs=[]  set_other_outputs_at_start=on  set_other_outputs_at_switch_in=off  set_other_outputs_at_terminate=on  set_other_outputs_at_switch_out=off  set_other_outputs_on_watchdog=off
  HIL Read : quarc_library/Data Acquisition/Generic/Immediate I//O/HIL Read  object_name=HIL-2  analog_channels=[5:6]  encoder_channels=[0]  digital_channels=[]  other_channels=[]  sample_time=qc_get_step_size  active=on  vector_output=off  data_type_mode=Inherit via back propagation  encoder_data_type=double  digital_data_type=boolean
  HIL Write : quarc_library/Data Acquisition/Generic/Immediate I//O/HIL Write  object_name=HIL-2  analog_channels=[]  pwm_channels=[0]  digital_channels=[40]  other_channels=[1000 11008:11011 11000:11003]  sample_time=qc_get_step_size  active=off  vector_input=on
  Mux : Mux  Inputs=2
  Scope : Scope  NumInputPorts=2
  Second-Order Low-Pass Filter : quarc_library/Continuous/Second-Order Low-Pass Filter  params_source=External (input ports)  input_width=1  input_zeta=1  input_init=0
  Second-Order Low-Pass Filter1 : quarc_library/Continuous/Second-Order Low-Pass Filter  params_source=External (input ports)  input_width=1  input_zeta=1  input_init=0
  Second-Order Low-Pass Filter2 : quarc_library/Continuous/Second-Order Low-Pass Filter  params_source=External (input ports)  input_width=1  input_zeta=1  input_init=0
  Steering Bias : Bias  Bias=0.0  SaturateOnIntegerOverflow=off
  Terminator : Terminator
  Terminator1 : Terminator
  Terminator2 : Terminator
  Unwrap 2^24 : quarc_library/Discontinuities/Inverse Modulus  modulus=16777215  output_derivative=off  output_revolutions=off  max_x=Inf  min_x=-Inf
  coast ON : Constant  Value=0
  command saturation : Saturate  UpperLimit=0.25  LowerLimit=-0.25
  direction convention : Gain  Gain=-1
  motorCurrent (A) [1] : Outport  VectorParamsAs1DForOutWhenUnconnected=off
  batteryVoltage (V) [1] : Outport  Port=2  VectorParamsAs1DForOutWhenUnconnected=off
  motorSpeed (counts/s) [1] : Outport  Port=3  VectorParamsAs1DForOutWhenUnconnected=off
  wires:
  Second-Order Low-Pass Filter2/1 -> Scope/1, motorCurrent (A) [1]/1  "battery voltage"
  Constant2/1 -> Second-Order Low-Pass Filter/2
  Unwrap 2^24/1 -> Second-Order Low-Pass Filter/4, Second-Order Low-Pass Filter/1
  Demux/2 -> Gain/1
  direction convention/1 -> command saturation/1
  "motorCmd (%, rad) [2]"/1 -> Demux/1
  command saturation/1 -> HIL Write/1
  Second-Order Low-Pass Filter/1 -> Terminator/1
  Constant3/1 -> Second-Order Low-Pass Filter1/3
  indicatorAndLamps (bool) [8]/1 -> Mux/2
  Steering Bias/1 -> Mux/1
  Second-Order Low-Pass Filter1/1 -> Scope/2, batteryVoltage (V) [1]/1  "battery voltage"
  Constant5/1 -> Second-Order Low-Pass Filter2/3
  Second-Order Low-Pass Filter1/2 -> Terminator1/1
  HIL Read/2 -> Second-Order Low-Pass Filter1/1, Second-Order Low-Pass Filter1/4  "battery voltage"
  Mux/1 -> HIL Write/3
  Constant6/1 -> Second-Order Low-Pass Filter2/2
  Second-Order Low-Pass Filter/2 -> motorSpeed (counts/s) [1]/1  "motor omega (counts/s)"
  Second-Order Low-Pass Filter2/2 -> Terminator2/1
  Constant4/1 -> Second-Order Low-Pass Filter1/2
  Constant1/1 -> Second-Order Low-Pass Filter/3
  Demux/1 -> direction convention/1
  HIL Read/3 -> Unwrap 2^24/1  "encoder counts"
  HIL Read/1 -> Second-Order Low-Pass Filter2/1, Second-Order Low-Pass Filter2/4  "motor current"
  Gain/1 -> Steering Bias/1
  coast ON/1 -> HIL Write/2

== system platoon1/QCar1/basicSpeedEstimation1 ==
  note: speedEstimation Module:
      |
      | This subsystem converts the motor speed measurements in counts/s to a useful longitudinal car speed in m/s.
      |
      | Inputs:
      | motorSpeed (counts/s) n/a : Drive motor speed measured using an encoder
      |
      | Outputs:
      | longitudinalCarSpeed (m/s) n/a : The platform's longitudinal speed (along the front-rear axis direction)
  note: (Diff. pinion*pinion)/(Spur*Diff. spur)
  note: v = 2*pi*r * omega (if omega is in rot/s)
      | v = r * omega (if omega is in rad/s)
      | r = 0.0342 m
  note: Estimate car speed from motor encoder counts rate
  motorSpeed (counts/s) : Inport
  counts to rotations : Gain  Gain=1/720/4
  gear ratios : Gain  Gain=(13*19)/(70*37)
  rot/s to rad/s : Gain  Gain=2*pi
  wheel radius : Gain  Gain=0.0342
  longitudinalCarSpeed (m/s) : Outport  VectorParamsAs1DForOutWhenUnconnected=off
  wires:
  gear ratios/1 -> rot/s to rad/s/1  "shaft speed (rots/s)"
  wheel radius/1 -> longitudinalCarSpeed (m/s)/1  "wheel speed (m/s)"
  counts to rotations/1 -> gear ratios/1  "motor speed (rot/s)"
  rot/s to rad/s/1 -> wheel radius/1  "wheel speed (rad/s)"
  motorSpeed (counts/s)/1 -> counts to rotations/1

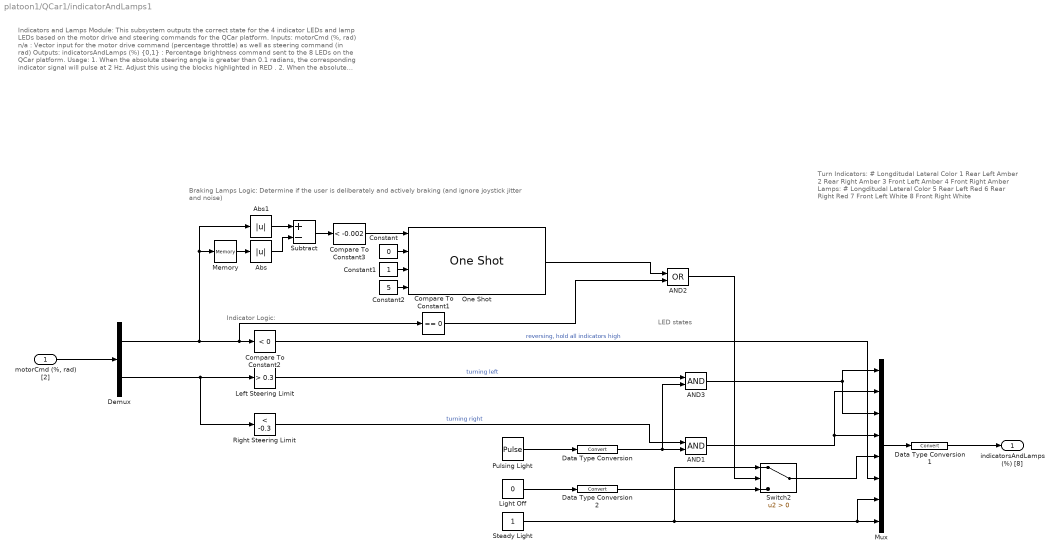
== system platoon1/QCar1/indicatorAndLamps1 ==
  note: Indicators and Lamps Module:
      |
      | This subsystem outputs the correct state for the 4 indicator LEDs and lamp LEDs based on the motor drive and steering commands for the QCar platform.
      |
      | Inputs:
      | motorCmd (%, rad) n/a : Vector input for the motor drive command (percentage throttle) as well as steering command (in rad)
      |
      | Outputs:
      | indicatorsAndLamps (%) {0,1} : Percentage brightness command sent to the 8 LEDs on the QCar platform.
      |
      | Usage:
      | 1. When the absolute steering angle is greater than 0.1 radians, the corresponding indicator signal will pulse at 2 Hz. Adjust this using the blocks highlighted in RED .
      | 2. When the absolute motor drive command approaches 0, the brake lamps will receive 100% brightness command, and 0% brightness otherwise. Adjust this using the blocks highlighted in GREEN .
  note: Braking Lamps Logic:
      | Determine if the user is deliberately and actively braking (and ignore joystick jitter and noise)
  note: LED states
  note: Turn Indicators:
      | # Longditudal Lateral Color
      | 1 Rear Left Amber
      | 2 Rear Right Amber
      | 3 Front Left Amber
      | 4 Front Right Amber
      |
      | Lamps:
      | # Longditudal Lateral Color
      | 5 Rear Left Red
      | 6 Rear Right Red
      | 7 Front Left White
      | 8 Front Right White
  note: Indicator Logic:
  "motorCmd (%, rad) [2]" : Inport
  AND1 : Logic  IconShape=distinctive  AllPortsSameDT=off  OutDataTypeStr=boolean
  AND2 : Logic  Operator=OR  IconShape=distinctive  AllPortsSameDT=off  OutDataTypeStr=boolean
  AND3 : Logic  IconShape=distinctive  AllPortsSameDT=off  OutDataTypeStr=boolean
  Abs : Abs  SaturateOnIntegerOverflow=off
  Abs1 : Abs  SaturateOnIntegerOverflow=off
  Compare To Constant1 : simulink/Logic and Bit Operations/Compare To Constant  relop===  const=0  OutDataTypeStr=uint8
  Compare To Constant2 : simulink/Logic and Bit Operations/Compare To Constant  relop=<  const=0  OutDataTypeStr=boolean
  Compare To Constant3 : simulink/Logic and Bit Operations/Compare To Constant  relop=<  const=-0.002  OutDataTypeStr=boolean
  Constant : Constant  Value=0
  Constant1 : Constant
  Constant2 : Constant  Value=5
  Data Type Conversion : DataTypeConversion  SaturateOnIntegerOverflow=off  RndMeth=Floor
  Data Type Conversion1 : DataTypeConversion  SaturateOnIntegerOverflow=off  RndMeth=Floor
  Data Type Conversion2 : DataTypeConversion  SaturateOnIntegerOverflow=off  RndMeth=Floor
  Demux : Demux  Outputs=2
  Left Steering Limit : simulink/Logic and Bit Operations/Compare To Constant  relop=>  const=0.3  OutDataTypeStr=boolean
  Light Off : Constant  Value=0  OutDataTypeStr=boolean
  Memory : Memory
  Mux : Mux  Inputs=8
  One Shot : quarc_library/Discontinuities/One Shot  trigger_type=Falling edge  redun_pulse=Ignore extraneous pulse  width_source=External input port  pulse_width=100
      settings: SourceProductName=QUARC Targets
  Pulsing Light : DiscretePulseGenerator  Period=0.5/qc_get_step_size  PulseWidth=0.5/2/qc_get_step_size  SampleTime=qc_get_step_size
  Right Steering Limit : simulink/Logic and Bit Operations/Compare To Constant  relop=<  const=-0.3  OutDataTypeStr=boolean
  Steady Light : Constant  OutDataTypeStr=boolean
  Subtract : Sum  Inputs=+-
  Switch2 : Switch  Criteria=u2 > Threshold  SaturateOnIntegerOverflow=off  InputSameDT=off
  indicatorsAndLamps (%) [8] : Outport  VectorParamsAs1DForOutWhenUnconnected=off
  wires:
  Data Type Conversion2/1 -> Switch2/3
  Demux/2 -> Right Steering Limit/1, Left Steering Limit/1
  Light Off/1 -> Data Type Conversion2/1
  One Shot/1 -> AND2/1
  Steady Light/1 -> Mux/7, Mux/8, Switch2/1
  Compare To Constant3/1 -> One Shot/1
  Constant2/1 -> One Shot/4
  Right Steering Limit/1 -> AND1/1  "turning right"
  Mux/1 -> Data Type Conversion1/1
  Constant/1 -> One Shot/2
  Pulsing Light/1 -> Data Type Conversion/1
  Abs/1 -> Subtract/2
  Memory/1 -> Abs/1
  Abs1/1 -> Subtract/1
  Data Type Conversion/1 -> AND3/2, AND1/2
  Data Type Conversion1/1 -> indicatorsAndLamps (%) [8]/1
  Left Steering Limit/1 -> AND3/1  "turning left"
  Switch2/1 -> Mux/5
  Constant1/1 -> One Shot/3
  Demux/1 -> Compare To Constant1/1, Compare To Constant2/1, Memory/1, Abs1/1
  AND3/1 -> Mux/1, Mux/3
  "motorCmd (%, rad) [2]"/1 -> Demux/1
  Subtract/1 -> Compare To Constant3/1
  AND1/1 -> Mux/2, Mux/4
  Compare To Constant2/1 -> Mux/6  "reversing, hold all indicators high"
  Compare To Constant1/1 -> AND2/2
  AND2/1 -> Switch2/2
